simulink model "etb_bosch"  (R2016a)
settings: Solver=ode15s  SolverMode=SingleTasking  StartTime=0.0  StopTime=2  RelTol=1e-3
libraries: fl_lib x11, nesl_utility x6, simulink x3, elec_lib x3, sh_lib x1
settings Model: Creator=Kevin  LastModifiedBy=ksheng
settings DebuggingCC: SFUnexpectedBacktrackingDiag=error  SFNoUnconditionalDefaultTransitionDiag=error
settings GRTTargetCC: TargetLangStandard=C99 (ISO)  GeneratePreprocessorConditionals=Use local settings
settings ConfigComp: CovMetricSettings=dwe  CovHtmlReporting=off  CovSaveCumulativeToWorkspaceVar=off  CovSaveSingleToWorkspaceVar=off  CovExternalEMLEnable=on

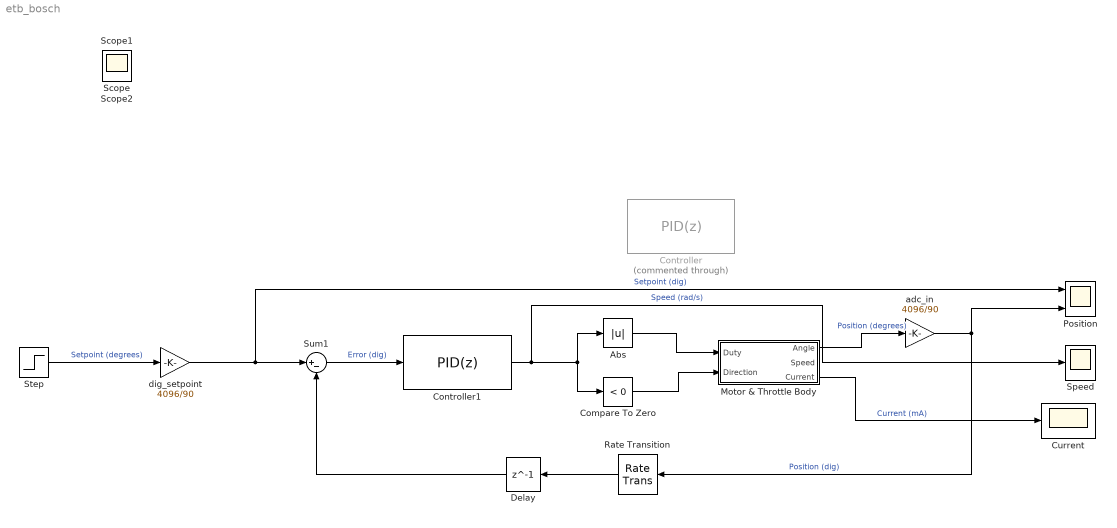
== system etb_bosch ==
  Abs : Abs
  Compare To Zero : simulink/Logic and Bit Operations/Compare To Zero  relop=<  OutDataTypeStr=uint8
  Controller : simulink/Continuous/PID Controller  Commented=through  Controller=PID  TimeDomain=Discrete-time  SampleTime=-1  IntegratorMethod=Forward Euler  FilterMethod=Forward Euler  Form=Parallel  UseFilter=on  ControllerParametersSource=internal  P=1.14275907316955  I=10.0776719941187  D=0  N=200  InitialConditionSource=internal  InitialConditionForIntegrator=0  InitialConditionForFilter=0  ExternalReset=none  LimitOutput=on  UpperSaturationLimit=100  LowerSaturationLimit=-100  LinearizeAsGain=off  AntiWindupMode=none  Kb=1  TrackingMode=off  Kt=1  PParamMin=[]  PParamMax=[]  IParamMin=[]  IParamMax=[]  DParamMin=[]  DParamMax=[]  NParamMin=[]  NParamMax=[]  KbParamMin=[]  KbParamMax=[]  KtParamMin=[]  KtParamMax=[]  POutMin=[]  POutMax=[]  IOutMin=[]  IOutMax=[]  DOutMin=[]  DOutMax=[]  NOutMin=[]  NOutMax=[]  KbOutMin=[]  KbOutMax=[]  KtOutMin=[]  KtOutMax=[]  IntegratorOutMin=[]  IntegratorOutMax=[]  FilterOutMin=[]  FilterOutMax=[]  SumOutMin=[]  SumOutMax=[]  SumI1OutMin=[]  SumI1OutMax=[]  SumI2OutMin=[]  SumI2OutMax=[]  SumI3OutMin=[]  SumI3OutMax=[]  SumDOutMin=[]  SumDOutMax=[]  SaturationOutMin=[]  SaturationOutMax=[]  IntegratorContinuousStateAttributes=''  IntegratorStateMustResolveToSignalObject=off  IntegratorRTWStateStorageClass=Auto  FilterContinuousStateAttributes=''  FilterStateMustResolveToSignalObject=off  FilterRTWStateStorageClass=Auto  DifferentiatorICPrevScaledInput=0  DifferentiatorOutMin=[]  DifferentiatorOutMax=[]
  Controller1 : simulink/Continuous/PID Controller  Controller=PID  TimeDomain=Discrete-time  SampleTime=-1  IntegratorMethod=Forward Euler  FilterMethod=Forward Euler  Form=Parallel  UseFilter=on  ControllerParametersSource=internal  P=0.177533835702716  I=1.438435490023  D=0.00390218818507904  N=218.373722092741  InitialConditionSource=internal  InitialConditionForIntegrator=0  InitialConditionForFilter=0  ExternalReset=none  LimitOutput=on  UpperSaturationLimit=50  LowerSaturationLimit=-50  LinearizeAsGain=off  AntiWindupMode=none  Kb=1  TrackingMode=off  Kt=1  PParamMin=[]  PParamMax=[]  IParamMin=[]  IParamMax=[]  DParamMin=[]  DParamMax=[]  NParamMin=[]  NParamMax=[]  KbParamMin=[]  KbParamMax=[]  KtParamMin=[]  KtParamMax=[]  POutMin=[]  POutMax=[]  IOutMin=[]  IOutMax=[]  DOutMin=[]  DOutMax=[]  NOutMin=[]  NOutMax=[]  KbOutMin=[]  KbOutMax=[]  KtOutMin=[]  KtOutMax=[]  IntegratorOutMin=[]  IntegratorOutMax=[]  FilterOutMin=[]  FilterOutMax=[]  SumOutMin=[]  SumOutMax=[]  SumI1OutMin=[]  SumI1OutMax=[]  SumI2OutMin=[]  SumI2OutMax=[]  SumI3OutMin=[]  SumI3OutMax=[]  SumDOutMin=[]  SumDOutMax=[]  SaturationOutMin=[]  SaturationOutMax=[]  IntegratorContinuousStateAttributes=''  IntegratorStateMustResolveToSignalObject=off  IntegratorRTWStateStorageClass=Auto  FilterContinuousStateAttributes=''  FilterStateMustResolveToSignalObject=off  FilterRTWStateStorageClass=Auto  DifferentiatorICPrevScaledInput=0  DifferentiatorOutMin=[]  DifferentiatorOutMax=[]
  Current : Scope
  Delay : Delay  DelayLength=1  InitialCondition=0
  Motor & Throttle Body : Subsystem
  Position : Scope  NumInputPorts=2
  Rate Transition : RateTransition  OutPortSampleTime=16e-6
  Speed : Scope
  Step : Step  After=5  SampleTime=1.6e-5
  Sum1 : Sum  Inputs=|+-
  adc_in : Gain  Gain=4096/90
  dig_setpoint : Gain  Gain=4096/90
  Scope : Scope
  Scope1 : Scope
  Scope2 : Scope
  wires:
  Sum1/1 -> Controller1/1  "Error (dig)"
  dig_setpoint/1 -> Position/1, Sum1/1  "Setpoint (dig)"
  adc_in/1 -> Rate Transition/1, Position/2  "Position (dig)"
  Rate Transition/1 -> Delay/1
  Abs/1 -> Motor & Throttle Body/1(Duty)
  Controller1/1 -> Speed/1, Abs/1, Compare To Zero/1  "Speed (rad/s)"
  Motor & Throttle Body/3(Current) -> Current/1  "Current (mA)"
  Compare To Zero/1 -> Motor & Throttle Body/2(Direction)
  Step/1 -> dig_setpoint/1  "Setpoint (degrees)"
  Motor & Throttle Body/1(Angle) -> adc_in/1  "Position (degrees)"
  Delay/1 -> Sum1/2

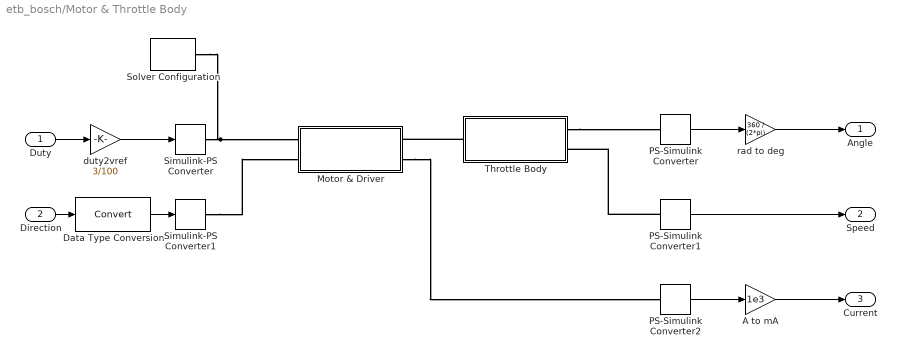
== system etb_bosch/Motor & Throttle Body ==
  Duty : Inport
  Direction : Inport  Port=2
  A to mA : Gain  Gain=1e3
  Data Type Conversion : DataTypeConversion
  Motor & Driver : Subsystem
  PS-Simulink Converter : nesl_utility/PS-Simulink Converter  PhysicalDomain=network_engine_domain  SubClassName=ps_output  LeftPortType=input  RightPortType=output  PseudoPeriodic=off  Frequencies=[]  Unit=1  AffineConversion=off
  PS-Simulink Converter1 : nesl_utility/PS-Simulink Converter  PhysicalDomain=network_engine_domain  SubClassName=ps_output  LeftPortType=input  RightPortType=output  PseudoPeriodic=off  Frequencies=[]  Unit=1  AffineConversion=off
  PS-Simulink Converter2 : nesl_utility/PS-Simulink Converter  PhysicalDomain=network_engine_domain  SubClassName=ps_output  LeftPortType=input  RightPortType=output  PseudoPeriodic=off  Frequencies=[]  Unit=1  AffineConversion=off
  Simulink-PS Converter : nesl_utility/Simulink-PS Converter  PhysicalDomain=network_engine_domain  SubClassName=ps_input  LeftPortType=input  RightPortType=output  PseudoPeriodic=off  Frequencies=[]  NoiseDistribution=none  NoiseParameters=[]  Unit=1  AffineConversion=off  InputFiltering=on  SimscapeFilterOrder=1  InputFilterTimeConstant=0.001  UdotUserProvided=1
  Simulink-PS Converter1 : nesl_utility/Simulink-PS Converter  PhysicalDomain=network_engine_domain  SubClassName=ps_input  LeftPortType=input  RightPortType=output  PseudoPeriodic=off  Frequencies=[]  NoiseDistribution=none  NoiseParameters=[]  Unit=1  AffineConversion=off  InputFiltering=on  SimscapeFilterOrder=1  InputFilterTimeConstant=0.001  UdotUserProvided=1
  Solver Configuration : nesl_utility/Solver Configuration  PhysicalDomain=network_engine_domain  SubClassName=solver  LeftPortType=input  RightPortType=generic  Accelerate=off  Tones=[]  Harmonics=[]  SimulateNoise=off  Profile=off  UseLocalSampling=off  EnableSwitchedLinearOptims=on  FrequencyDomain=off  UseCCode=off  RelTol=0.001  AbsTol=1e-06  MinStep=1e-09  ToWorkspace=off  RevertToSquareIcSolve=off  NumHomotopyIterations=100  PhasorMode=off  PhasorModeNumHarmonics=1  OverrideAbsTol=off  DoDC=off  ResidualTolerance=1e-09  UseLocalSolver=off  LocalSolverChoice=NE_BACKWARD_EULER_ADVANCER  LocalSolverSampleTime=0.001  DoFixedCost=off  MaxNonlinIter=3  MaxModeIter=2  LinearAlgebra=Sparse  DelaysMemoryBudget=1024  AutomaticFiltering=on  FilteringTimeConstant=0.001
  Throttle Body : Subsystem
  duty2vref : Gain  Gain=3/100
  rad to deg : Gain  Gain=360 / (2*pi)
  Angle : Outport
  Speed : Outport  Port=2
  Current : Outport  Port=3
  wires:
  Duty/1 -> duty2vref/1
  PS-Simulink Converter/1 -> rad to deg/1
  rad to deg/1 -> Angle/1
  PS-Simulink Converter1/1 -> Speed/1
  PS-Simulink Converter2/1 -> A to mA/1
  A to mA/1 -> Current/1
  duty2vref/1 -> Simulink-PS Converter/1
  Direction/1 -> Data Type Conversion/1
  Data Type Conversion/1 -> Simulink-PS Converter1/1
  connections:
  Simulink-PS Converter/RConn1 -- Solver Configuration/RConn1 -- Motor & Driver/LConn1
  Throttle Body/RConn1 -- PS-Simulink Converter/LConn1
  Throttle Body/LConn1 -- Motor & Driver/RConn1
  Simulink-PS Converter1/RConn1 -- Motor & Driver/LConn2
  PS-Simulink Converter1/LConn1 -- Throttle Body/RConn2
  Motor & Driver/RConn2 -- PS-Simulink Converter2/LConn1

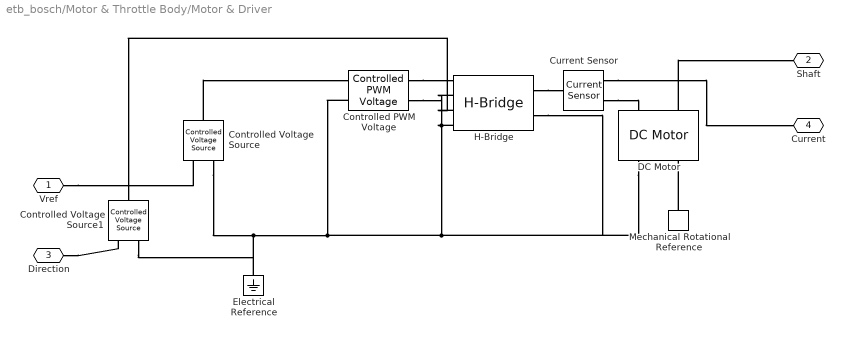
== system etb_bosch/Motor & Throttle Body/Motor & Driver ==
  Controlled Voltage Source : fl_lib/Electrical/Electrical Sources/Controlled Voltage Source
  Controlled Voltage Source1 : fl_lib/Electrical/Electrical Sources/Controlled Voltage Source
  Controlled PWM Voltage : elec_lib/Actuators & Drivers/Drivers/Controlled PWM Voltage  F=20 kHz  TD=0 s  pulse_width_offset=0 s  Vmin=0 V  Vmax=3 V  Vm=6 V  pwm_or_av=2  event_type=1  sample_time=1e-6 s
  Current Sensor : fl_lib/Electrical/Electrical Sensors/Current Sensor
  DC Motor : elec_lib/Actuators & Drivers/Rotational Actuators/DC Motor  parameterization=2  Ra=2.5 Ohm  La=.0211 H  emf_or_torque=2  Kv=.084 V/rpm  Ki=6.876e-4 N*m/A  T_stall=.23303 N*m  w_max=290 rpm  w_rated=1.5e+4 rpm  P_rated=0.08 W  V_rated=6 V  J=3.1321e-6 kg*m^2  lam_param=2  lam=1e-06 N*m/(rad/s)  i_noload=250 mA  V_i_noload=6 V  speed0=0 rpm  alpha=0.00393 1/K  Tmeas=25 degC  thermal_mass=100 J/K  initial_temperature=25 degC
  Electrical Reference : fl_lib/Electrical/Electrical Elements/Electrical Reference
  H-Bridge : elec_lib/Actuators & Drivers/Drivers/H-Bridge  Venable=2.5 V  Vmax=6 V  Vreverse=.1 V  Vbrake=2.5 V  Vm=6 V  pwm_or_av=2  discontinuous=0  freewheeling_mode=1  freewheeling_mode_disc=1  Ron=0.1 Ohm  Don=0.05 Ohm  Rload=10 Ohm  Lload=1e-5 H  F=10 kHz  thermal_mass=100 J/K  initial_temperature=298.15 K  Ron2=0.1 Ohm  Don2=0.05 Ohm  Tmeas=298.15 K  Tmeas2=398.15 K
  Mechanical Rotational Reference : fl_lib/Mechanical/Rotational Elements/Mechanical Rotational Reference
  Vref : PMIOPort  Port=1  Side=Left
  Shaft : PMIOPort  Port=2  Side=Right
  Direction : PMIOPort  Port=3  Side=Left
  Current : PMIOPort  Port=4  Side=Right
  connections:
  Mechanical Rotational Reference/LConn1 -- DC Motor/RConn2
  Vref/RConn1 -- Controlled Voltage Source/RConn1
  Controlled Voltage Source/RConn2 -- Controlled Voltage Source1/RConn2 -- Electrical Reference/LConn1 -- Controlled PWM Voltage/RConn2 -- H-Bridge/LConn2 -- H-Bridge/LConn4 -- DC Motor/RConn1 -- H-Bridge/RConn2 -- Controlled PWM Voltage/LConn2
  Controlled Voltage Source/LConn1 -- Controlled PWM Voltage/LConn1
  Controlled PWM Voltage/RConn1 -- H-Bridge/LConn1
  Direction/RConn1 -- Controlled Voltage Source1/RConn1
  H-Bridge/LConn3 -- Controlled Voltage Source1/LConn1
  DC Motor/LConn2 -- Shaft/RConn1
  H-Bridge/RConn1 -- Current Sensor/LConn1
  Current Sensor/RConn2 -- DC Motor/LConn1
  Current Sensor/RConn1 -- Current/RConn1

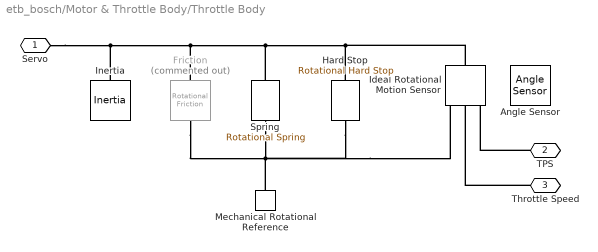
== system etb_bosch/Motor & Throttle Body/Throttle Body ==
  Angle Sensor : sh_lib/Pumps and Motors/Angle Sensor  phase_angle=0 rad
  Friction : fl_lib/Mechanical/Rotational Elements/Rotational Friction  Commented=on  brkwy_trq=.19 * .75 / 12 lbf*ft  Col_trq=.19 * .75 / 12 lbf*ft  visc_coef=0 N*m/(rad/s)  trans_coef=10 s/rad  vel_thr=1e-4 rad/s  w_specify=off  w_priority=None  w=0 rad/s  t_specify=off  t_priority=None  t=0 N*m
  Hard Stop : fl_lib/Mechanical/Rotational Elements/Rotational Hard Stop  upper_bnd=90 deg  lower_bnd=0 deg  stiff_up=1e6 N*m/rad  stiff_low=1e6 N*m/rad  D_up=0.01 N*m/(rad/s)  D_low=0.01 N*m/(rad/s)  w_specify=off  w_priority=None  w=0 rad/s  t_specify=off  t_priority=None  t=0 N*m  phi_specify=off  phi_priority=High  phi=0 rad
  Ideal Rotational Motion Sensor : fl_lib/Mechanical/Mechanical Sensors/Ideal Rotational Motion Sensor  offset=0 rad
  Inertia : fl_lib/Mechanical/Rotational Elements/Inertia  inertia=.01 lbm*in^2  w_specify=off  w_priority=High  w=0 rad/s  t_specify=off  t_priority=None  t=0 N*m
  Mechanical Rotational Reference : fl_lib/Mechanical/Rotational Elements/Mechanical Rotational Reference
  Spring : fl_lib/Mechanical/Rotational Elements/Rotational Spring  spr_rate=.230 in*lbf/deg  w_specify=off  w_priority=None  w=0 rad/s  t_specify=off  t_priority=None  t=0 N*m  phi_specify=off  phi_priority=High  phi=0 rad
  "Servo " : PMIOPort  Port=1  Side=Left
  TPS : PMIOPort  Port=2  Side=Right
  Throttle Speed : PMIOPort  Port=3  Side=Right
  connections:
  Inertia/LConn1 -- "Servo "/RConn1 -- Friction/LConn1 -- Spring/LConn1 -- Ideal Rotational Motion Sensor/LConn1 -- Hard Stop/LConn1
  TPS/RConn1 -- Ideal Rotational Motion Sensor/RConn3
  Spring/RConn1 -- Friction/RConn1 -- Ideal Rotational Motion Sensor/RConn1 -- Hard Stop/RConn1 -- Mechanical Rotational Reference/LConn1
  Throttle Speed/RConn1 -- Ideal Rotational Motion Sensor/RConn2
